simulink model "PD_INDI_flightController"  (R2021b)
settings: Solver=VariableStepAuto  StartTime=0.0  StopTime=10.0  RelTol=1e-3
settings Model: Creator=Tiga  LastModifiedBy=Tiga

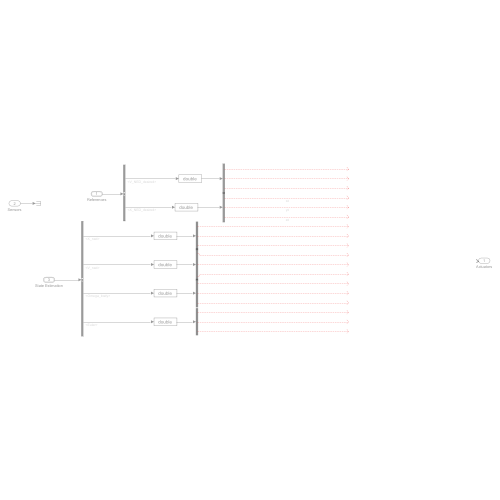
[thumbnail: Simulink's stored preview of the top-level diagram]
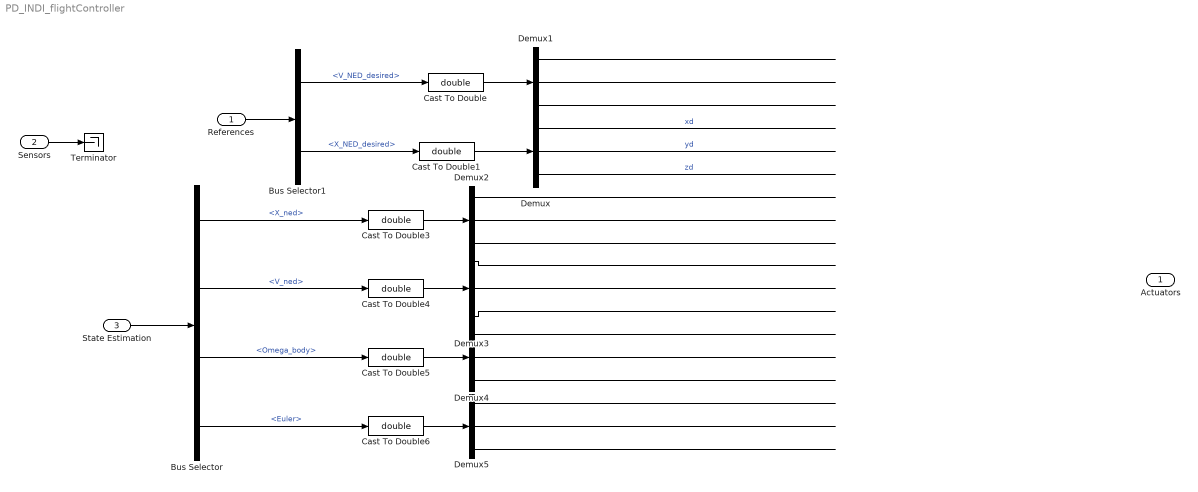
== system PD_INDI_flightController ==
  References : Inport  OutDataTypeStr=Bus: ReferencesBus
  Sensors : Inport  Port=2
  State Estimation : Inport  Port=3  OutDataTypeStr=Bus: StatesBus
  Bus Selector : BusSelector  OutputSignals=X_ned,V_ned,Omega_body,Euler
  Bus Selector1 : BusSelector  OutputSignals=V_NED_desired,X_NED_desired
  Cast To Double{,1,3..6} (6 alike) : DataTypeConversion  OutDataTypeStr=double
  Demux{,1..5} (6 alike) : Demux  Outputs=3
  Terminator : Terminator
  Actuators : Outport
  wires:
  Bus Selector1/1 -> Cast To Double/1  "<V_NED_desired>"
  Sensors/1 -> Terminator/1
  Demux2/3 -> ?
  Demux3/2 -> ?
  Demux4/1 -> ?
  Demux3/1 -> ?
  Demux/1 -> ?  "xd"
  References/1 -> Bus Selector1/1
  Demux/2 -> ?  "yd"
  Demux5/3 -> ?
  Demux4/3 -> ?
  Bus Selector/4 -> Cast To Double6/1  "<Euler>"
  Demux5/1 -> ?
  State Estimation/1 -> Bus Selector/1
  Cast To Double5/1 -> Demux4/1
  Bus Selector/3 -> Cast To Double5/1  "<Omega_body>"
  Demux1/2 -> ?
  Bus Selector1/2 -> Cast To Double1/1  "<X_NED_desired>"
  Demux1/3 -> ?
  Cast To Double/1 -> Demux1/1
  Demux3/3 -> ?
  Demux1/1 -> ?
  Demux5/2 -> ?
  Cast To Double6/1 -> Demux5/1
  Demux2/2 -> ?
  Bus Selector/2 -> Cast To Double4/1  "<V_ned>"
  Cast To Double1/1 -> Demux/1
  Cast To Double4/1 -> Demux3/1
  Demux/3 -> ?  "zd"
  Cast To Double3/1 -> Demux2/1
  Bus Selector/1 -> Cast To Double3/1  "<X_ned>"
  Demux4/2 -> ?
  Demux2/1 -> ?
